simulink model "exampleStorage_type2_hx_fintube_strat"  (Simulink 7.6)
settings: Solver=ode45  StartTime=0.0  StopTime=3*3600-2  RelTol=1e-3
libraries: carnot x15, simulink x4
settings Model: Creator=drhf  LastModifiedBy=drhf
settings CodeAppCC: CustomSymbolStrType=$N$R$M_T

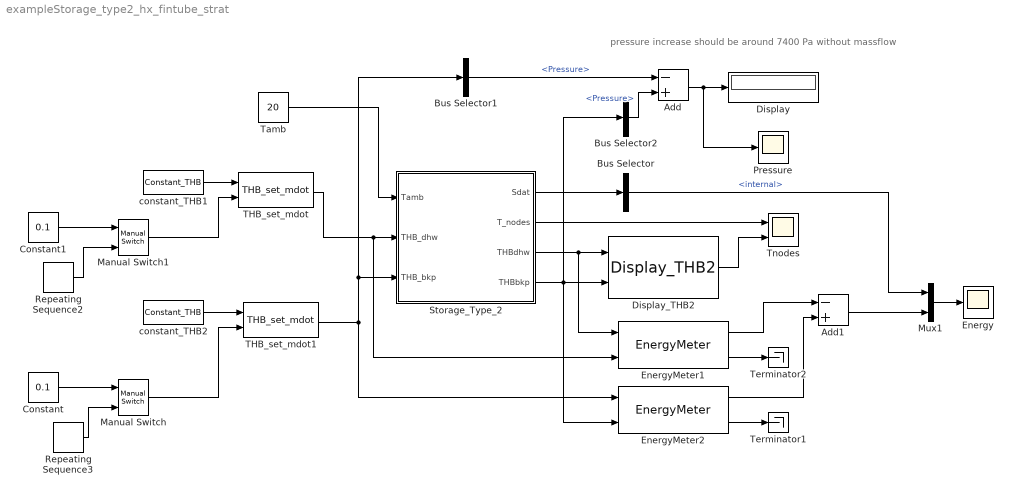
== system exampleStorage_type2_hx_fintube_strat ==
  note: pressure increase should be around 7400 Pa without massflow
  Add : Sum  Inputs=-+
  Add1 : Sum  Inputs=-+
  Bus Selector : BusSelector  OutputSignals=energy.internal
  Bus Selector1 : BusSelector  OutputSignals=Pressure
  Bus Selector2 : BusSelector  OutputSignals=Pressure
  Constant : Constant  Value=0.1
  Constant1 : Constant  Value=0.1
  Display : Display
  Display_THB2 : carnot/Outputs/Display_THB2  SystemSampleTime=-1  t=off  m=on  p=off  id=off  mix=off  d=off
  Energy : Scope
  EnergyMeter1 : carnot/Control/EnergyMeter  SystemSampleTime=-1
  EnergyMeter2 : carnot/Control/EnergyMeter  SystemSampleTime=-1
  Manual Switch : simulink/Signal Routing/Manual Switch  SystemSampleTime=-1  sw=0  action=0  varsize=off
  Manual Switch1 : simulink/Signal Routing/Manual Switch  SystemSampleTime=-1  sw=0  action=0  varsize=off
  Mux1 : Mux  Inputs=2
  Pressure : Scope
  Repeating Sequence2 : simulink/Sources/Repeating Sequence  SystemSampleTime=-1  rep_seq_t=[0 1 1 2 2 2.9 2.9 3.1]*3600  rep_seq_y=[0.0 0.0 0.15 0.15 0.1 0.1 0 0]
  Repeating Sequence3 : simulink/Sources/Repeating Sequence  SystemSampleTime=-1  rep_seq_t=[0 1 1 2 2 3]*3600  rep_seq_y=[0.12 0.12 0.1 0.1 0.15 0.15]
  Storage_Type_2 : Subsystem  mask(Multiport Storage){uloss=1, ubot=1, utop=1, cond=1, tini=[20:5:65], volume=0.3, dia=0.5, pos=standing cylinder, nconnect=2, nodes=10, mpoints=10}
      mask prompts: uloss "Heat loss coefficient cylinder wall in W/(m²K)"; ubot "Heat loss coefficient bottom in W/(m²K)"; utop "Heat loss coefficient top cover in W/(m²K)"; cond "Effective vertical conductivity in W/(m*K)"; tini "Initial temperature (vector or scalar) in °C"; volume "Volume in m³"; dia "Diameter in m"; pos "Position"; nconnect "Number of connections"; nodes "Number of nodes"; mpoints "Number of measurement points"
      mask help:
      | The volmue of the cylindrical storage is divided in a number "nodes" of horizontal slices (1xN-node model). For each node the energy balance equation is solved.
      | Look under mask to set the ports types and properties.
      mask init:
      | standing = pos-1;
      | 
      | if standing
      |     dh = volume/(0.25*dia^2*pi*nodes);
      | else
      |     dh = dia/nodes;
      | end
      | 
      | height = dh*nodes;
      | 
      | mpoints = max(mpoints,1);
      | mpts = round(nodes/mpoints/2:nodes/mpoints:nodes);
      mask Help: eval('man(''storage_multiport'')')
      mask StyleString: edit,edit,edit,edit,edit,edit,edit,popup(lying cylinder|standing cylinder),edit,edit,edit
      mask TabNameString: Thermal,Thermal,Thermal,Thermal,Thermal,Geometry,Geometry,Geometry,Geometry,Calculation,Calculation
      mask Display: plot(10,20,80,100,[36,36,40,50,54,54,50,40,36],[90,50,45,45,50,90,93,93,90],[36,51,44,51,36],[50,50,55,60,60])
  THB_set_mdot : carnot/Source/Simple/THB_set_mdot  SystemSampleTime=-1
  THB_set_mdot1 : carnot/Source/Simple/THB_set_mdot  SystemSampleTime=-1
  Tamb : Constant  Value=20
  Terminator1 : Terminator
  Terminator2 : Terminator
  Tnodes : Scope  NumInputPorts=2
      settings: YMin=-5~-5  YMax=5~5  SaveName=ScopeData3
  constant_THB1 : carnot/Source/Simple/Constant_THB  SystemSampleTime=-1  t=10  mdot=0*100/3600  p=1e5  mID=Full Pressure Drop with Static Height  fluid=water  mix=0  dia=0.02  hgt=0
  constant_THB2 : carnot/Source/Simple/Constant_THB  SystemSampleTime=-1  t=55  mdot=100/3600  p=1e5  mID=Full Pressure Drop with Static Height  fluid=water  mix=0  dia=0.02  hgt=0
  wires:
  Bus Selector/1 -> Mux1/1  "<internal>"
  Tamb/1 -> Storage_Type_2/1(Tamb)
  THB_set_mdot/1 -> Storage_Type_2/2(THB_dhw), EnergyMeter1/2
  THB_set_mdot1/1 -> Storage_Type_2/3(THB_bkp), Bus Selector1/1, EnergyMeter2/1
  Storage_Type_2/1(Sdat) -> Bus Selector/1
  Storage_Type_2/2(T_nodes) -> Tnodes/1
  Storage_Type_2/3(THBdhw) -> EnergyMeter1/1, Display_THB2/1
  Storage_Type_2/4(THBbkp) -> Bus Selector2/1, EnergyMeter2/2, Display_THB2/2
  Display_THB2/1 -> Tnodes/2
  Mux1/1 -> Energy/1
  EnergyMeter2/2 -> Terminator1/1
  Add/1 -> Display/1, Pressure/1
  Bus Selector1/1 -> Add/1  "<Pressure>"
  Bus Selector2/1 -> Add/2  "<Pressure>"
  EnergyMeter1/2 -> Terminator2/1
  Add1/1 -> Mux1/2
  EnergyMeter2/1 -> Add1/2
  EnergyMeter1/1 -> Add1/1
  constant_THB1/1 -> THB_set_mdot/1
  constant_THB2/1 -> THB_set_mdot1/1
  Manual Switch1/1 -> THB_set_mdot/2
  Manual Switch/1 -> THB_set_mdot1/2
  Constant/1 -> Manual Switch/1
  Repeating Sequence3/1 -> Manual Switch/2
  Constant1/1 -> Manual Switch1/1
  Repeating Sequence2/1 -> Manual Switch1/2

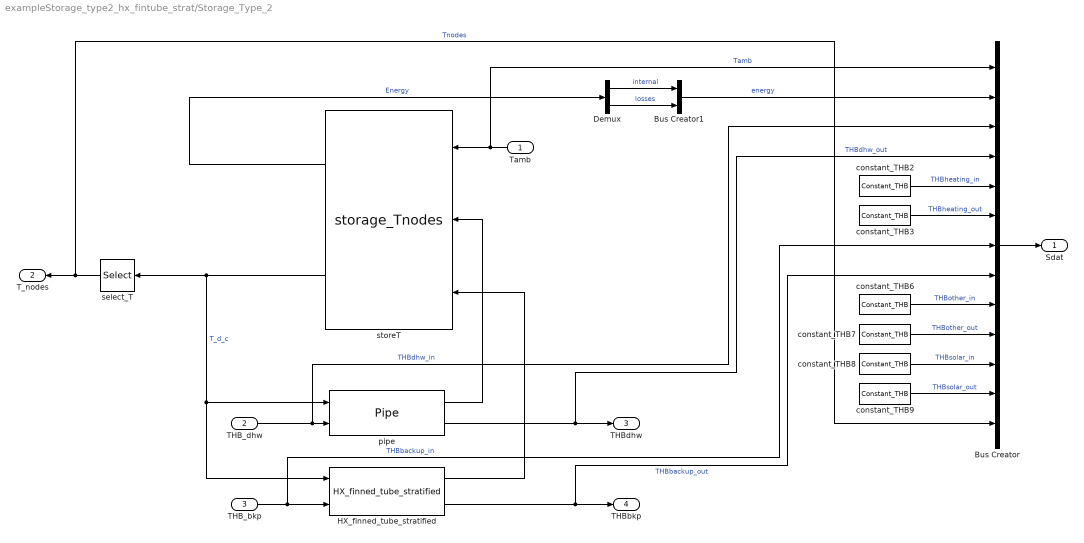
== system exampleStorage_type2_hx_fintube_strat/Storage_Type_2 ==
  Tamb : Inport
  THB_dhw : Inport  Port=2
  THB_bkp : Inport  Port=3
  Bus Creator : BusCreator  Inputs=13
  Bus Creator1 : BusCreator  Inputs=2
  Demux : Demux  Outputs=2
  HX_finned_tube_stratified : carnot/Storage/Thermal/Storage_Ports/HX_finned_tube_stratified  SystemSampleTime=-1  h_in=1  h_out=0  dpipe=0.03  swall=0.002  lpipe=15  cond=50  dfin=0.05  sfin=0.001  nfin=100  dplin=100  dpqua=100  nodes=nodes  hgt=height  dia=dia
  constant_THB{2..3,6..9} (6 alike) : carnot/Source/Simple/Constant_THB  SystemSampleTime=-1  t=20  mdot=0  p=1e5  mID=No Pressure Drop  fluid=water  mix=0  dia=0.02  hgt=0
  pipe : carnot/Storage/Thermal/Storage_Ports/Pipe  SystemSampleTime=-1  h_in=0  h_out=1  dplin=0  dpqua=0  nodes=nodes  hgt=height  dia=dia
  select_T : Selector  InputPortWidth=nodes  IndexOptions=Index vector (dialog)  Indices=mpts  OutputSizes=1
  storeT : S-Function  FunctionName=storage_Tnodes  Parameters=dia, volume, standing, uloss , ubot, utop, cond, tini, nodes, nconnect  EnableBusSupport=off
  Sdat : Outport
  T_nodes : Outport  Port=2
  THBdhw : Outport  Port=3
  THBbkp : Outport  Port=4
  wires:
  Tamb/1 -> storeT/1, Bus Creator/1  "Tamb"
  THB_dhw/1 -> Bus Creator/3, pipe/2  "THBdhw_in"
  pipe/2 -> Bus Creator/4, THBdhw/1  "THBdhw_out"
  pipe/1 -> storeT/2
  select_T/1 -> T_nodes/1, Bus Creator/13  "Tnodes"
  storeT/1 -> Demux/1  "Energy"
  storeT/2 -> select_T/1, pipe/1, HX_finned_tube_stratified/1  "T_d_c"
  Bus Creator/1 -> Sdat/1
  constant_THB9/1 -> Bus Creator/12  "THBsolar_out"
  constant_THB8/1 -> Bus Creator/11  "THBsolar_in"
  constant_THB7/1 -> Bus Creator/10  "THBother_out"
  constant_THB6/1 -> Bus Creator/9  "THBother_in"
  constant_THB2/1 -> Bus Creator/5  "THBheating_in"
  constant_THB3/1 -> Bus Creator/6  "THBheating_out"
  THB_bkp/1 -> Bus Creator/7, HX_finned_tube_stratified/2  "THBbackup_in"
  HX_finned_tube_stratified/2 -> Bus Creator/8, THBbkp/1  "THBbackup_out"
  HX_finned_tube_stratified/1 -> storeT/3
  Demux/1 -> Bus Creator1/1  "internal"
  Demux/2 -> Bus Creator1/2  "losses"
  Bus Creator1/1 -> Bus Creator/2  "energy"
